simulink model "mbackprop1"  (Simulink 6.3)
settings: Solver=ode5  StartTime=0.0  StopTime=30  RelTol=1e-3
PreLoadFcn:
  | load mdlref_counter_bus.mat
settings Model: Creator=The MathWorks Inc.  LastModifiedBy=mshakeri  ExtModeAutoUpdateStatusClock=off  StrictBusMsg=ErrorLevel1
settings DataIOCC: SignalLoggingName=logsOut
settings OptimizationCC: InlineParams=on  InlineInvariantSignals=on  BufferReusableBoundary=off
settings DebuggingCC: CheckExecutionContextPreStartOutputMsg=on  CheckExecutionContextRuntimeOutputMsg=on  SolverPrmCheckMsg=none  BusObjectLabelMismatch=error
settings HardwareCC: TargetHWDeviceType=32-bit Generic
settings ModelReferenceCC: UpdateModelReferenceTargets=IfOutOfDate
settings RTWCC: GenerateReport=on  ProcessScript=grt_make_rtw_hook  LaunchReport=on

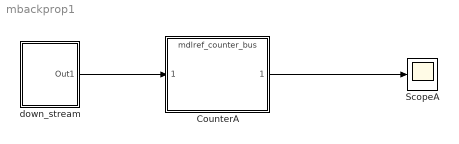
== system mbackprop1 ==
  CounterA : ModelReference  ModelName=mdlref_counter_bus  ModelReferenceVersion=1.114  CopyOfModelName=mdlref_counter_bus
  ScopeA : Scope
      settings: TimeRange=30  YMax=50  SaveName=ScopeDataA  DataFormat=Array
  down_stream : Subsystem  TreatAsAtomicUnit=on
  wires:
  down_stream/1(Out1) -> CounterA/1
  CounterA/1 -> ScopeA/1

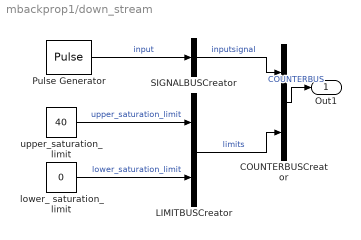
== system mbackprop1/down_stream ==
  COUNTERBUSCreator : BusCreator  Inputs=2
  LIMITBUSCreator : BusCreator  Inputs=2
  Pulse Generator : DiscretePulseGenerator  Amplitude=int32(1)  SampleTime=0.1
  SIGNALBUSCreator : BusCreator  Inputs=1
  lower_ saturation_ limit : Constant  Value=0  OutDataTypeMode=int32  SampleTime=0.1
  upper_saturation_limit : Constant  Value=40  OutDataTypeMode=int32  SampleTime=0.1
  Out1 : Outport
  wires:
  upper_saturation_limit/1 -> LIMITBUSCreator/1  "upper_saturation_limit"
  lower_ saturation_ limit/1 -> LIMITBUSCreator/2  "lower_saturation_limit"
  LIMITBUSCreator/1 -> COUNTERBUSCreator/2  "limits"
  Pulse Generator/1 -> SIGNALBUSCreator/1  "input"
  SIGNALBUSCreator/1 -> COUNTERBUSCreator/1  "inputsignal"
  COUNTERBUSCreator/1 -> Out1/1  "COUNTERBUS"
